simulink model "p_4"  (R2020b)
settings: Solver=VariableStepAuto  StartTime=0.0  StopTime=20.0  RelTol=1e-3
values from neighbouring files (symbols this model uses):
  A1 = 3    [P_4.m]
  A2 = 5    [P_4.m]
  g = 32.2    [P_4.m]
  h1 = 2    [P_4.m]
  h2 = 5    [P_4.m]
  R1 = 30    [P_4.m]
  rho = 1.94    [P_4.m]
settings Model: Creator=Tiankuo  LastModifiedBy=Tiankuo

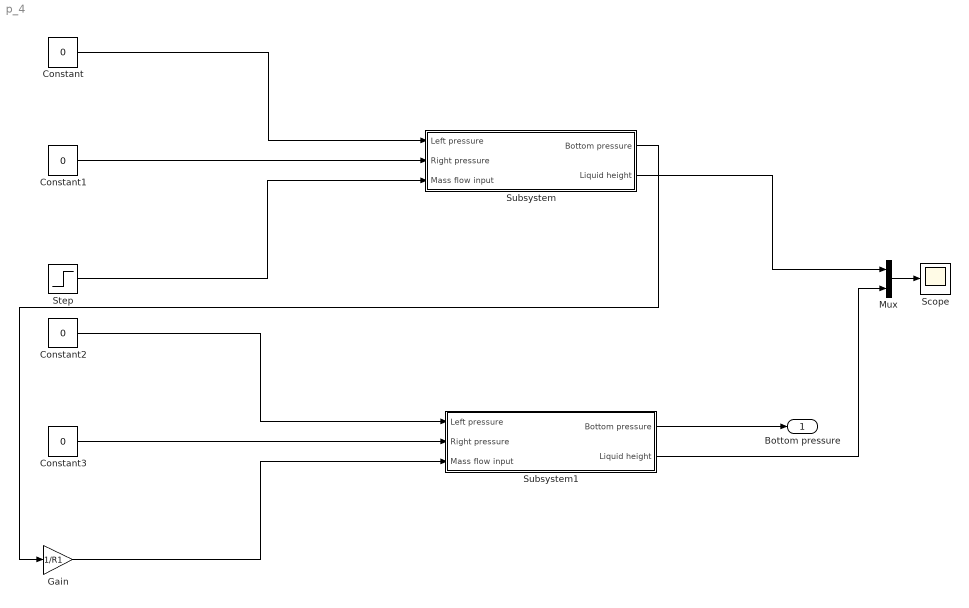
== system p_4 ==
  Constant{,1..3} (4 alike) : Constant  Value=0
  Gain : Gain  Gain=1/R1
  Mux : Mux  Inputs=2
  Scope : Scope
  Step : Step  After=0.5  SampleTime=0
  Subsystem : Subsystem
  Subsystem1 : Subsystem
  Bottom pressure : Outport
  wires:
  Constant/1 -> Subsystem/1(Left pressure)
  Constant1/1 -> Subsystem/2(Right pressure)
  Step/1 -> Subsystem/3(Mass flow input)
  Subsystem1/1(Bottom pressure) -> Bottom pressure/1
  Gain/1 -> Subsystem1/3(Mass flow input)
  Constant3/1 -> Subsystem1/2(Right pressure)
  Constant2/1 -> Subsystem1/1(Left pressure)
  Subsystem1/2(Liquid height) -> Mux/2
  Mux/1 -> Scope/1
  Subsystem/2(Liquid height) -> Mux/1
  Subsystem/1(Bottom pressure) -> Gain/1

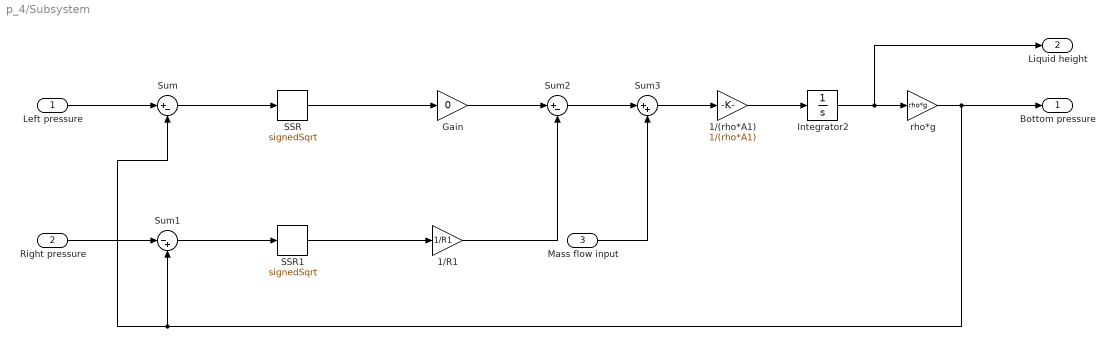
== system p_4/Subsystem ==
  Left pressure : Inport
  Right pressure : Inport  Port=2
  Mass flow input : Inport  Port=3
  1/(rho*A1) : Gain  Gain=1/(rho*A1)
  1/R1 : Gain  Gain=1/R1
  Gain : Gain  Gain=0
  Integrator2 : Integrator  InitialCondition=h1
  SSR : Sqrt  Operator=signedSqrt  SaturateOnIntegerOverflow=on
  SSR1 : Sqrt  Operator=signedSqrt  SaturateOnIntegerOverflow=on
  Sum : Sum  Inputs=|+-
  Sum1 : Sum  Inputs=|-+
  Sum2 : Sum  Inputs=|+-
  Sum3 : Sum  Inputs=|++
  rho*g : Gain  Gain=rho*g
  Bottom pressure : Outport
  Liquid height : Outport  Port=2
  wires:
  Sum/1 -> SSR/1
  Sum2/1 -> Sum3/1
  Sum1/1 -> SSR1/1
  Integrator2/1 -> Liquid height/1, rho*g/1
  SSR/1 -> Gain/1
  Mass flow input/1 -> Sum3/2
  rho*g/1 -> Bottom pressure/1, Sum/2, Sum1/2
  Left pressure/1 -> Sum/1
  1/R1/1 -> Sum2/2
  Right pressure/1 -> Sum1/1
  SSR1/1 -> 1/R1/1
  Gain/1 -> Sum2/1
  1/(rho*A1)/1 -> Integrator2/1
  Sum3/1 -> 1/(rho*A1)/1

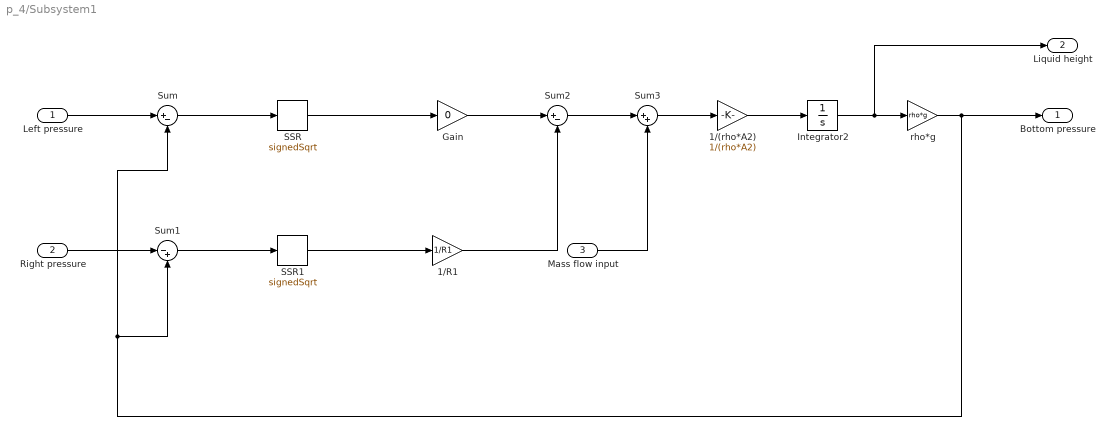
== system p_4/Subsystem1 ==
  Left pressure : Inport
  Right pressure : Inport  Port=2
  Mass flow input : Inport  Port=3
  1/(rho*A2) : Gain  Gain=1/(rho*A2)
  1/R1 : Gain  Gain=1/R1
  Gain : Gain  Gain=0
  Integrator2 : Integrator  InitialCondition=h2
  SSR : Sqrt  Operator=signedSqrt  SaturateOnIntegerOverflow=on
  SSR1 : Sqrt  Operator=signedSqrt  SaturateOnIntegerOverflow=on
  Sum : Sum  Inputs=|+-
  Sum1 : Sum  Inputs=|-+
  Sum2 : Sum  Inputs=|+-
  Sum3 : Sum  Inputs=|++
  rho*g : Gain  Gain=rho*g
  Bottom pressure : Outport
  Liquid height : Outport  Port=2
  wires:
  Sum/1 -> SSR/1
  Sum2/1 -> Sum3/1
  Sum1/1 -> SSR1/1
  Integrator2/1 -> Liquid height/1, rho*g/1
  SSR/1 -> Gain/1
  Mass flow input/1 -> Sum3/2
  rho*g/1 -> Bottom pressure/1, Sum/2, Sum1/2
  Left pressure/1 -> Sum/1
  1/R1/1 -> Sum2/2
  Right pressure/1 -> Sum1/1
  SSR1/1 -> 1/R1/1
  Gain/1 -> Sum2/1
  1/(rho*A2)/1 -> Integrator2/1
  Sum3/1 -> 1/(rho*A2)/1
